simulink model "VFU_PhaseLack"  (Simulink 7.9)
settings: Solver=ode45  StartTime=0.0  StopTime=10  RelTol=1e-3
libraries: powerlib x33, powerlib_extras x1
settings Model: Creator=H002220  LastModifiedBy=H002220

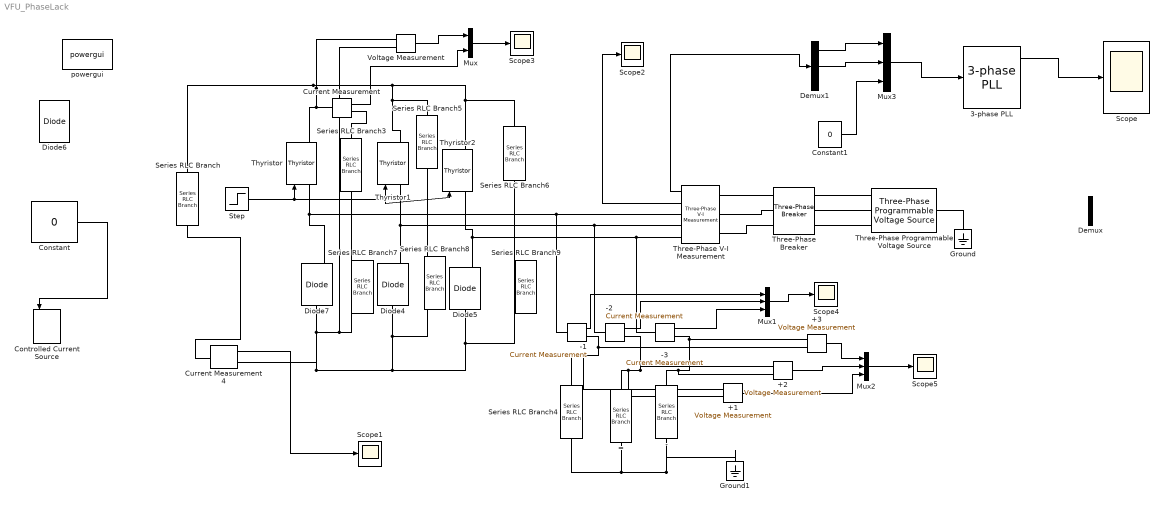
== system VFU_PhaseLack ==
  +1 : powerlib/Measurements/Voltage Measurement  PhasorSimulation=off  OutputType=Complex  PSBequivalent=0
  +2 : powerlib/Measurements/Voltage Measurement  PhasorSimulation=off  OutputType=Complex  PSBequivalent=0
  +3 : powerlib/Measurements/Voltage Measurement  PhasorSimulation=off  OutputType=Complex  PSBequivalent=0
  - : powerlib/Elements/Series RLC Branch  LConnTagsString=__new0  RConnTagsString=__new0  BranchType=C  Resistance=0.02  Inductance=1e-3  SetiL0=off  InitialCurrent=0  Capacitance=1e-6  Setx0=off  InitialVoltage=0  Measurements=None
  -1 : powerlib/Measurements/Current Measurement  PhasorSimulation=off  OutputType=Complex  PSBequivalent=0
  -2 : powerlib/Measurements/Current Measurement  PhasorSimulation=off  OutputType=Complex  PSBequivalent=0
  -3 : powerlib/Measurements/Current Measurement  PhasorSimulation=off  OutputType=Complex  PSBequivalent=0
  3-phase PLL : powerlib_extras/Control  Blocks/3-phase PLL  Par_Init=[0 60]  ParK=[ 220 22200 1 ]  AGC=off
  = : powerlib/Elements/Series RLC Branch  LConnTagsString=__new0  RConnTagsString=__new0  BranchType=C  Resistance=0.02  Inductance=1e-3  SetiL0=off  InitialCurrent=0  Capacitance=1e-6  Setx0=off  InitialVoltage=0  Measurements=None
  Constant : Constant  Value=0
  Constant1 : Constant  Value=0
  Controlled Current Source : powerlib/Electrical Sources/Controlled Current Source  Initialize=on  Source_Type=AC  Amplitude=0  Phase=0  Frequency=0  Measurements=None
  Current Measurement : powerlib/Measurements/Current Measurement  PhasorSimulation=off  OutputType=Complex  PSBequivalent=0
  Current Measurement4 : powerlib/Measurements/Current Measurement  PhasorSimulation=off  OutputType=Complex  PSBequivalent=0
  Demux : Demux  Outputs=2
  Demux1 : Demux  Outputs=3
  Diode{4..7} (4 alike) : powerlib/Power Electronics/Diode  Ron=0.001  Lon=0  Vf=0.8  IC=0  UseSnubber=off  Rs=500  Cs=250e-9  Measurements=on
  Ground : powerlib/Elements/Ground  LConnTagsString=a
  Ground1 : powerlib/Elements/Ground  LConnTagsString=a
  Mux : Mux  Inputs=2
  Mux1 : Mux  Inputs=3
  Mux2 : Mux  Inputs=3
  Mux3 : Mux  Inputs=3
  Scope{,1..5} (6 alike) : Scope
      Scope2 settings: SaveName=ScopeData2
      Scope3 settings: SaveName=ScopeData3
      Scope4 settings: SaveName=ScopeData4
      Scope5 settings: SaveName=ScopeData5
  Series RLC Branch : powerlib/Elements/Series RLC Branch  LConnTagsString=__new0  RConnTagsString=__new0  BranchType=C  Resistance=1  Inductance=20e-3  SetiL0=on  InitialCurrent=12  Capacitance=600e-6  Setx0=on  InitialVoltage=500  Measurements=None
  Series RLC Branch3 : powerlib/Elements/Series RLC Branch  LConnTagsString=__new0  RConnTagsString=__new0  BranchType=RC  Resistance=8  Inductance=1e-3  SetiL0=off  InitialCurrent=0  Capacitance=0.33e-6  Setx0=off  InitialVoltage=0  Measurements=None
  Series RLC Branch4 : powerlib/Elements/Series RLC Branch  LConnTagsString=__new0  RConnTagsString=__new0  BranchType=C  Resistance=1  Inductance=1e-3  SetiL0=off  InitialCurrent=0  Capacitance=1e-6  Setx0=off  InitialVoltage=0  Measurements=None
  Series RLC Branch5 : powerlib/Elements/Series RLC Branch  LConnTagsString=__new0  RConnTagsString=__new0  BranchType=RC  Resistance=8  Inductance=1e-3  SetiL0=off  InitialCurrent=0  Capacitance=0.33e-6  Setx0=off  InitialVoltage=0  Measurements=None
  Series RLC Branch6 : powerlib/Elements/Series RLC Branch  LConnTagsString=__new0  RConnTagsString=__new0  BranchType=RC  Resistance=8  Inductance=1e-3  SetiL0=off  InitialCurrent=0  Capacitance=0.33e-6  Setx0=off  InitialVoltage=0  Measurements=None
  Series RLC Branch7 : powerlib/Elements/Series RLC Branch  LConnTagsString=__new0  RConnTagsString=__new0  BranchType=RC  Resistance=1  Inductance=1e-3  SetiL0=off  InitialCurrent=0  Capacitance=1e-6  Setx0=off  InitialVoltage=0  Measurements=None
  Series RLC Branch8 : powerlib/Elements/Series RLC Branch  LConnTagsString=__new0  RConnTagsString=__new0  BranchType=RC  Resistance=1  Inductance=1e-3  SetiL0=off  InitialCurrent=0  Capacitance=1e-6  Setx0=off  InitialVoltage=0  Measurements=None
  Series RLC Branch9 : powerlib/Elements/Series RLC Branch  LConnTagsString=__new0  RConnTagsString=__new0  BranchType=RC  Resistance=1  Inductance=1e-3  SetiL0=off  InitialCurrent=0  Capacitance=1e-6  Setx0=off  InitialVoltage=0  Measurements=None
  Step : Step  Time=0.025  Before=1  After=0  SampleTime=0
  Three-Phase Programmable Voltage Source : powerlib/Electrical Sources/Three-Phase Programmable Voltage Source  PositiveSequence="[380  0 50]"  VariationEntity=None  VariationType=Table of time-amplitude pairs  VariationTypeAlt=Step  VariationStep=0.5  VariationRate=10  VariationMagnitude=0.3  VariationFrequency=2  VariationTiming=[1 2]  VariationPhaseA=off  Amplitudes=[1 0.8 1.2 1.0]  TimeValues=[0 0.1 0.15 0.2]  HarmonicGeneration=off  HarmonicA=[3 0.2 -25 0]  HarmonicB=[2 0.15 35 2]  Timing="[0.05  3]"  BusType=swing  Pref=0  Qref=0  Qmin=-inf  Qmax=inf
  Three-Phase V-I Measurement : powerlib/Measurements/Three-Phase V-I Measurement  VoltageMeasurement=phase-to-ground  SetLabelV=off  LabelV=Vabc  Vpu=off  VpuLL=off  CurrentMeasurement=yes  SetLabelI=off  LabelI=Iabc  Ipu=off  Pbase=100e6  Vbase=500e3  OutputType=Complex  PhasorSimulation=off  PSBequivalent=0
  Three-Phase Breaker : powerlib/Elements/Three-Phase Breaker  InitialState=closed  SwitchA=on  SwitchB=on  SwitchC=on  SwitchTimes=[2]  External=off  BreakerResistance=0.001  SnubberResistance=1e6  SnubberCapacitance=inf  Measurements=None
  Thyristor : powerlib/Power Electronics/Thyristor  Ron=0.001  Lon=0  Vf=0.8  IC=0  Rs=500  Cs=250e-9  Measurements=on
  Thyristor1 : powerlib/Power Electronics/Thyristor  Ron=0.001  Lon=0  Vf=0.8  IC=0  Rs=500  Cs=250e-9  Measurements=on
  Thyristor2 : powerlib/Power Electronics/Thyristor  Ron=0.001  Lon=0  Vf=0.8  IC=0  Rs=500  Cs=250e-9  Measurements=on
  Voltage Measurement : powerlib/Measurements/Voltage Measurement  PhasorSimulation=off  OutputType=Complex  PSBequivalent=0
  powergui : powerlib/powergui  Priority=1  SimulationMode=Discrete  SolverType=Backward Euler  SampleTime=50e-6  frequency=60  SPID=off  DisableSnubberDevices=off  DisableRonSwitches=off  DisableVfSwitches=off  SwTol=0  Interpol=off  DisplayEquations=off  FunctionMessages=off  frequencyindice=50  Pbase=100e6  ErrMax=1e-4  Iterations=50  UnitsV=kV  UnitsW=MW  echomessages=off  HookPort=off  EnableUseOfTLC=off  x0status=blocks  RestoreLinks=warning  ResistiveCurrentMeasurement=off  Ylog=off  Xlog=on  ShowGrid=off  save=off  variable=ZData  ZoomFFT=off  StartTime=0.0  cycles=1  DisplayStyle=1  FreqAxis=off  MaxFrequency=1000  frequencyindicesteady=1  display=off  methode=off
  wires:
  Current Measurement4/1 -> Scope1/1
  Constant/1 -> Controlled Current Source/1
  Three-Phase V-I Measurement/1 -> Demux1/1
  Three-Phase V-I Measurement/2 -> Scope2/1
  Voltage Measurement/1 -> Mux/1
  Current Measurement/1 -> Mux/2
  Mux/1 -> Scope3/1
  -1/1 -> Mux1/1
  -2/1 -> Mux1/2
  -3/1 -> Mux1/3
  +3/1 -> Mux2/1
  +2/1 -> Mux2/2
  +1/1 -> Mux2/3
  Mux1/1 -> Scope4/1
  Mux2/1 -> Scope5/1
  Step/1 -> Thyristor/1, Thyristor1/1, Thyristor2/1
  Demux1/1 -> Mux3/1
  Demux1/2 -> Mux3/2
  Constant1/1 -> Mux3/3
  Mux3/1 -> 3-phase PLL/1
  3-phase PLL/1 -> Scope/1
  connections:
  Ground/LConn1 -- Three-Phase Programmable Voltage Source/LConn1
  Diode5/LConn1 -- Current Measurement4/RConn1 -- Diode7/LConn1 -- Series RLC Branch3/RConn1 -- Voltage Measurement/LConn2 -- Diode4/LConn1 -- Series RLC Branch5/RConn1 -- Series RLC Branch6/RConn1
  Thyristor2/RConn1 -- Voltage Measurement/LConn1 -- Current Measurement/LConn1 -- Thyristor/RConn1 -- Series RLC Branch/LConn1 -- Series RLC Branch5/LConn1 -- Thyristor1/RConn1 -- Series RLC Branch6/LConn1
  Thyristor1/LConn1 -- Three-Phase V-I Measurement/RConn2 -- -2/LConn1 -- Diode4/RConn1
  Thyristor2/LConn1 -- Three-Phase V-I Measurement/RConn3 -- -3/LConn1 -- Diode5/RConn1
  Series RLC Branch/RConn1 -- Current Measurement4/LConn1
  Ground1/LConn1 -- Series RLC Branch4/RConn1 -- =/RConn1 -- -/RConn1
  Three-Phase Programmable Voltage Source/RConn1 -- Three-Phase Breaker/LConn1
  Three-Phase Programmable Voltage Source/RConn2 -- Three-Phase Breaker/LConn2
  Three-Phase Programmable Voltage Source/RConn3 -- Three-Phase Breaker/LConn3
  Three-Phase Breaker/RConn1 -- Three-Phase V-I Measurement/LConn1
  Three-Phase Breaker/RConn2 -- Three-Phase V-I Measurement/LConn2
  Three-Phase Breaker/RConn3 -- Three-Phase V-I Measurement/LConn3
  Current Measurement/RConn1 -- Series RLC Branch3/LConn1
  Series RLC Branch4/LConn1 -- +1/LConn1 -- -1/RConn1 -- +3/LConn2
  -2/RConn1 -- +2/LConn1 -- =/LConn1 -- +1/LConn2
  -/LConn1 -- +2/LConn2 -- -3/RConn1 -- +3/LConn1
  Diode7/RConn1 -- Three-Phase V-I Measurement/RConn1 -- -1/LConn1 -- Thyristor/LConn1
